simulink model "MUX"  (R2019b)
settings: Solver=VariableStepAuto  StartTime=0.0  StopTime=4  RelTol=1e-3
libraries: hdlsllib x3
settings Model: Creator=cohen  LastModifiedBy=cohen

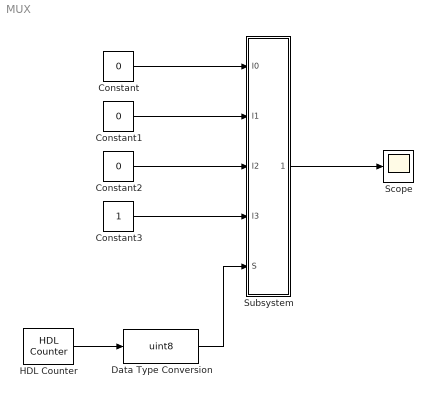
== system MUX ==
  Constant : Constant  Value=0  OutDataTypeStr=boolean
  Constant1 : Constant  Value=0  OutDataTypeStr=boolean
  Constant2 : Constant  Value=0  OutDataTypeStr=boolean
  Constant3 : Constant  OutDataTypeStr=boolean
  Data Type Conversion : DataTypeConversion  OutDataTypeStr=uint8
  HDL Counter : hdlsllib/Sources/HDL Counter  CountType=Free running  CountInit=0  CountStep=1  CountMax=25  CountFromType=Initial value  CountFrom=0  CountResetPort=off  CountLoadPort=off  CountEnbPort=off  CountDirPort=off  CountDataType=Unsigned  CountWordLen=2  CountFracLen=0  CountSampTime=1
      settings: SourceProductName=Simulink
  Scope : Scope
  Subsystem : Subsystem
  wires:
  Constant/1 -> Subsystem/1(I0)
  Constant1/1 -> Subsystem/2(I1)
  Constant2/1 -> Subsystem/3(I2)
  Constant3/1 -> Subsystem/4(I3)
  Subsystem/1(Out1) -> Scope/1
  HDL Counter/1 -> Data Type Conversion/1
  Data Type Conversion/1 -> Subsystem/5(S)

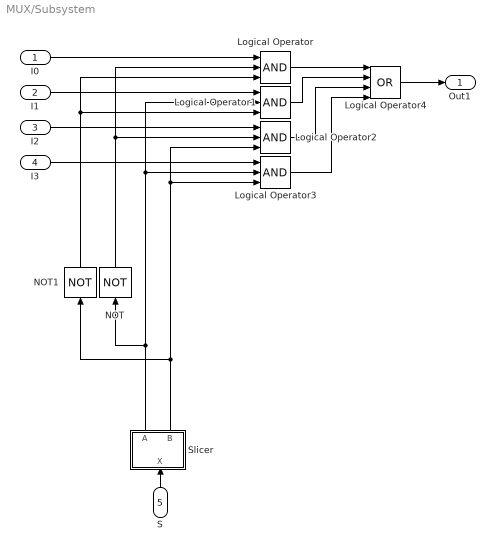
== system MUX/Subsystem ==
  I0 : Inport
  I1 : Inport  Port=2
  I2 : Inport  Port=3
  I3 : Inport  Port=4
  S : Inport  Port=5  OutDataTypeStr=uint8
  Logical Operator{,1..3} (4 alike) : Logic  Inputs=3  AllPortsSameDT=off  OutDataTypeStr=boolean
  Logical Operator4 : Logic  Operator=OR  Inputs=4  AllPortsSameDT=off  OutDataTypeStr=boolean
  NOT : Logic  Operator=NOT  IconShape=distinctive  AllPortsSameDT=off  OutDataTypeStr=boolean
  NOT1 : Logic  Operator=NOT  IconShape=distinctive  AllPortsSameDT=off  OutDataTypeStr=boolean
  Slicer : Subsystem
  Out1 : Outport
  wires:
  Logical Operator1/1 -> Logical Operator4/2
  NOT/1 -> Logical Operator/2, Logical Operator2/2
  I1/1 -> Logical Operator1/1
  I2/1 -> Logical Operator2/1
  NOT1/1 -> Logical Operator/3, Logical Operator1/3
  I3/1 -> Logical Operator3/1
  I0/1 -> Logical Operator/1
  Logical Operator2/1 -> Logical Operator4/3
  Logical Operator4/1 -> Out1/1
  Logical Operator3/1 -> Logical Operator4/4
  Logical Operator/1 -> Logical Operator4/1
  S/1 -> Slicer/1(X)
  Slicer/2(B) -> NOT1/1, Logical Operator2/3, Logical Operator3/3
  Slicer/1(A) -> NOT/1, Logical Operator1/2, Logical Operator3/2

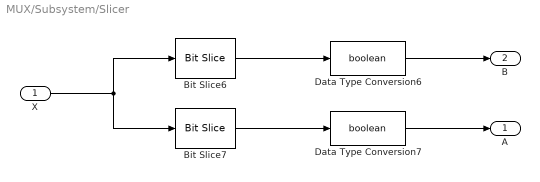
== system MUX/Subsystem/Slicer ==
  X : Inport  OutDataTypeStr=uint8  SampleTime=1
  Bit Slice6 : hdlsllib/Logic and Bit Operations/Bit Slice  lidx=1  ridx=1
      settings: SourceProductName=Simulink  SourceProductBaseCode=SL
  Bit Slice7 : hdlsllib/Logic and Bit Operations/Bit Slice  lidx=0  ridx=0
      settings: SourceProductName=Simulink  SourceProductBaseCode=SL
  Data Type Conversion6 : DataTypeConversion  OutDataTypeStr=boolean
  Data Type Conversion7 : DataTypeConversion  OutDataTypeStr=boolean
  A : Outport  OutDataTypeStr=boolean  SampleTime=1
  B : Outport  Port=2  OutDataTypeStr=boolean  SampleTime=1
  wires:
  Bit Slice6/1 -> Data Type Conversion6/1
  X/1 -> Bit Slice6/1, Bit Slice7/1
  Bit Slice7/1 -> Data Type Conversion7/1
  Data Type Conversion7/1 -> A/1
  Data Type Conversion6/1 -> B/1
